simulink model "hostpc_can"  (Simulink 7.3)
settings: Solver=VariableStepDiscrete  StartTime=0.0  StopTime=inf  RelTol=1e-3
libraries: simulink x33, amg_usbconverter_n_connect_lib x3
settings Model: Creator=Nav  LastModifiedBy=Nav

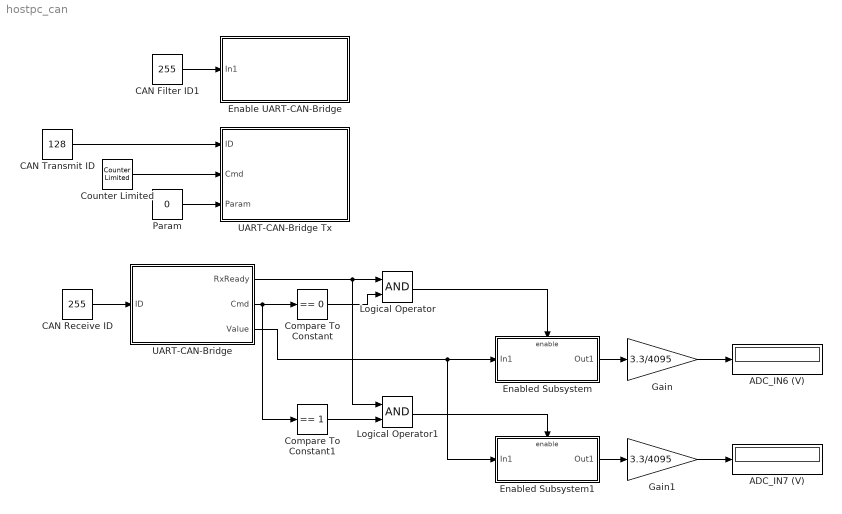
== system hostpc_can ==
  ADC_IN6 (V) : Display
  ADC_IN7 (V) : Display
  CAN Filter ID1 : Constant  Value=255  OutDataTypeMode=uint32  OutDataType=fixdt(1, 16)  OutScaling=2^0  OutDataTypeStr=uint32
  CAN Receive ID : Constant  Value=255  OutDataTypeMode=uint32  OutDataType=fixdt(1, 16)  OutScaling=2^0  OutDataTypeStr=uint32
  CAN Transmit ID : Constant  Value=128  OutDataTypeMode=uint32  OutDataType=fixdt(1, 16)  OutScaling=2^0  OutDataTypeStr=uint32
  Compare To Constant : simulink/Logic and Bit Operations/Compare To Constant  SystemSampleTime=-1  relop===  const=0  LogicOutDataTypeMode=boolean  ZeroCross=off
  Compare To Constant1 : simulink/Logic and Bit Operations/Compare To Constant  SystemSampleTime=-1  relop===  const=1  LogicOutDataTypeMode=boolean  ZeroCross=off
  Counter Limited : simulink/Sources/Counter Limited  SystemSampleTime=-1  uplimit=1  tsamp=-1
  Enable UART-CAN-Bridge : Subsystem  Priority=0
  Enabled Subsystem : Subsystem  TreatAsAtomicUnit=on
  Enabled Subsystem1 : Subsystem  TreatAsAtomicUnit=on
  Gain : Gain  Gain=3.3/4095  ParameterDataType=fixdt(1, 16)  ParameterScaling=2^0  OutDataType=fixdt(1, 16)  OutScaling=2^0
  Gain1 : Gain  Gain=3.3/4095  ParameterDataType=fixdt(1, 16)  ParameterScaling=2^0  OutDataType=fixdt(1, 16)  OutScaling=2^0
  Logical Operator : Logic  AllPortsSameDT=off  OutDataTypeMode=boolean  LogicDataType=fixdt(0, 8)  OutDataTypeStr=boolean
  Logical Operator1 : Logic  AllPortsSameDT=off  OutDataTypeMode=boolean  LogicDataType=fixdt(0, 8)  OutDataTypeStr=boolean
  Param : Constant  Value=0  OutDataTypeMode=uint32  OutDataType=fixdt(1, 16)  OutScaling=2^0  OutDataTypeStr=uint32
  UART-CAN-Bridge : Subsystem  Priority=2
  UART-CAN-Bridge Tx : Subsystem  Priority=1
  wires:
  CAN Receive ID/1 -> UART-CAN-Bridge/1(ID)
  CAN Transmit ID/1 -> UART-CAN-Bridge Tx/1(ID)
  Counter Limited/1 -> UART-CAN-Bridge Tx/2(Cmd)
  Param/1 -> UART-CAN-Bridge Tx/3(Param)
  UART-CAN-Bridge/2(Cmd) -> Compare To Constant/1, Compare To Constant1/1
  UART-CAN-Bridge/1(RxReady) -> Logical Operator/1, Logical Operator1/1
  Compare To Constant/1 -> Logical Operator/2
  Logical Operator/1 -> Enabled Subsystem/Enable
  UART-CAN-Bridge/3(Value) -> Enabled Subsystem/1(In1), Enabled Subsystem1/1(In1)
  Enabled Subsystem/1(Out1) -> Gain/1
  Logical Operator1/1 -> Enabled Subsystem1/Enable
  Compare To Constant1/1 -> Logical Operator1/2
  Enabled Subsystem1/1(Out1) -> Gain1/1
  CAN Filter ID1/1 -> Enable UART-CAN-Bridge/1(In1)
  Gain/1 -> ADC_IN6 (V)/1
  Gain1/1 -> ADC_IN7 (V)/1

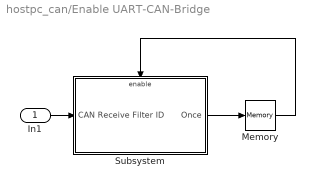
== system hostpc_can/Enable UART-CAN-Bridge ==
  In1 : Inport
  Memory : Memory  X0=1  InheritSampleTime=on  LinearizeMemory=on
  Subsystem : Subsystem
  wires:
  Subsystem/1(Once) -> Memory/1
  Memory/1 -> Subsystem/Enable
  In1/1 -> Subsystem/1(CAN Receive Filter ID)

== system hostpc_can/Enabled Subsystem ==
  In1 : Inport  OutDataType=fixdt(1, 16)  OutScaling=2^0
  Enable : EnablePort
  Out1 : Outport  OutDataType=fixdt(1, 16)  OutScaling=2^0
  wires:
  In1/1 -> Out1/1

== system hostpc_can/Enabled Subsystem1 ==
  In1 : Inport  OutDataType=fixdt(1, 16)  OutScaling=2^0
  Enable : EnablePort
  Out1 : Outport  OutDataType=fixdt(1, 16)  OutScaling=2^0
  wires:
  In1/1 -> Out1/1

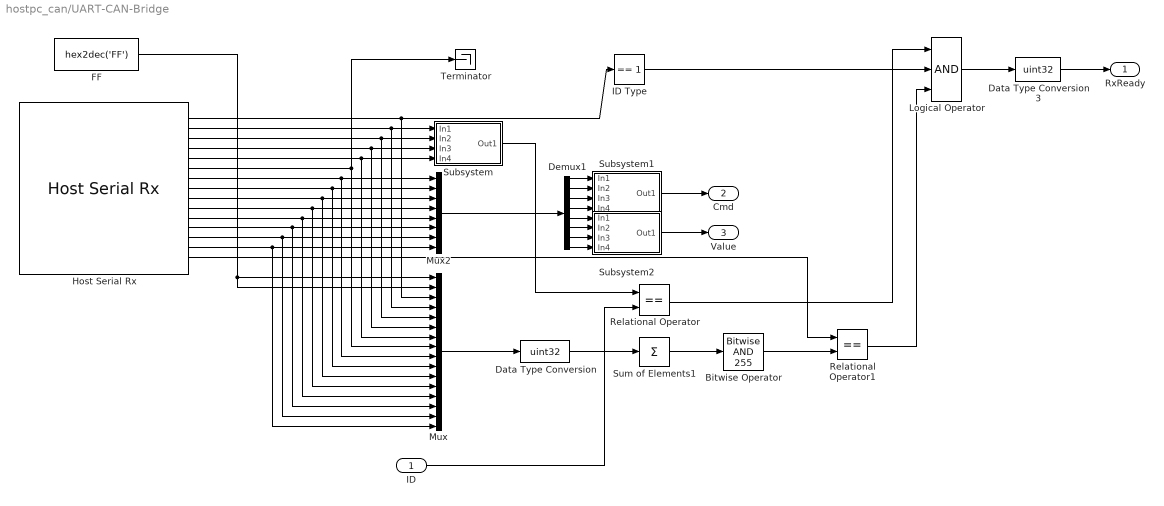
== system hostpc_can/UART-CAN-Bridge ==
  ID : Inport  OutDataType=fixdt(1, 16)  OutScaling=2^0
  Bitwise Operator : simulink/Logic and Bit Operations/Bitwise Operator  logicop=AND  UseBitMask=on  BitMask=255  BitMaskRealWorld=Stored Integer
  Data Type Conversion : DataTypeConversion  OutDataTypeMode=uint32  OutDataType=fixdt(1, 16)  OutScaling=2^0  OutDataTypeStr=uint32
  Data Type Conversion3 : DataTypeConversion  OutDataTypeMode=uint32  OutDataType=fixdt(1, 16)  OutScaling=2^0  OutDataTypeStr=uint32
  Demux1 : Demux  Outputs=8
  FF : Constant  Value=hex2dec('FF')  OutDataTypeMode=uint8  OutDataType=fixdt(1, 16)  OutScaling=2^0  OutDataTypeStr=uint8
  Host Serial Rx : amg_usbconverter_n_connect_lib/Host Serial Rx  conf=rx  port=<auto>  baudrate=115200  databits=8  parity=None  stopbit=1  flowcontrol=None  transfer=Blocking  timeout=2  packetmode=Binary  initialvalues=[0]  binheader='FF FF'  binterminator=''  porttype_double=0  porttype_single=0  porttype_int8=0  porttype_uint8=15  porttype_int16=0  porttype_uint16=0  porttype_int32=0  porttype_uint32=0  asciiformat='%d %u %x'  rx_asciiterminator="CRLF (0x0D 0x0A - \"\\r\\n\")"  tx_asciiterminator="CRLF (0x0D 0x0A - \"\\r\\n\")"  sampletime=inf  enablecustomportlabel=off  cinputportlabel=0  coutputportlabel=A  portpinstr=0  blockid=UARTCANBridgeHostSerialRx  inputporttype=[]  inputportwidth=[]  inputportlabel={}  outputporttype=[3 3 3 3 3 3 3 3 3 3 3 3 3 3 3]  outputportwidth=[1 1 1 1 1 1 1 1 1 1 1 1 1 1 1]  outputportlabel={'uint8','uint8','uint8','uint8','uint8','uint8','uint8','uint8','uint8','uint8','uint8','uint8','uint8','uint8','uint8'}  compat=0  optionstring="[\"Param1\",\"Param1\"]"  autoport='COM3'
  ID Type : simulink/Logic and Bit Operations/Compare To Constant  SystemSampleTime=-1  relop===  const=1  LogicOutDataTypeMode=uint8  ZeroCross=off
  Logical Operator : Logic  Inputs=3  AllPortsSameDT=off  OutDataTypeMode=boolean  LogicDataType=fixdt(0, 8)  OutDataTypeStr=boolean
  Mux : Mux  Inputs=16
  Mux2 : Mux  Inputs=8
  Relational Operator : RelationalOperator  Operator===  LogicOutDataTypeMode=boolean  LogicDataType=fixdt(0, 8)  OutDataTypeStr=boolean
  Relational Operator1 : RelationalOperator  Operator===  LogicOutDataTypeMode=boolean  LogicDataType=fixdt(0, 8)  OutDataTypeStr=boolean
  Subsystem : Subsystem
  Subsystem1 : Subsystem
  Subsystem2 : Subsystem
  Sum of Elements1 : Sum  Inputs=+  OutDataType=fixdt(1, 16)  OutScaling=2^-10
  Terminator : Terminator
  RxReady : Outport
  Cmd : Outport  Port=2
  Value : Outport  Port=3
  wires:
  Sum of Elements1/1 -> Bitwise Operator/1
  Host Serial Rx/15 -> Relational Operator1/1
  Mux/1 -> Data Type Conversion/1
  FF/1 -> Mux/2, Mux/1
  Subsystem/1(Out1) -> Relational Operator/1
  ID/1 -> Relational Operator/2
  Logical Operator/1 -> Data Type Conversion3/1
  Mux2/1 -> Demux1/1
  ID Type/1 -> Logical Operator/2
  Data Type Conversion/1 -> Sum of Elements1/1
  Bitwise Operator/1 -> Relational Operator1/2
  Host Serial Rx/1 -> ID Type/1, Mux/3
  Host Serial Rx/2 -> Subsystem/1(In1), Mux/4
  Host Serial Rx/3 -> Subsystem/2(In2), Mux/5
  Host Serial Rx/4 -> Subsystem/3(In3), Mux/6
  Host Serial Rx/5 -> Subsystem/4(In4), Mux/7
  Host Serial Rx/6 -> Terminator/1, Mux/8
  Host Serial Rx/7 -> Mux2/1, Mux/9
  Host Serial Rx/8 -> Mux2/2, Mux/10
  Host Serial Rx/9 -> Mux2/3, Mux/11
  Host Serial Rx/10 -> Mux2/4, Mux/12
  Host Serial Rx/11 -> Mux2/5, Mux/13
  Host Serial Rx/12 -> Mux2/6, Mux/14
  Host Serial Rx/13 -> Mux2/7, Mux/15
  Host Serial Rx/14 -> Mux2/8, Mux/16
  Relational Operator/1 -> Logical Operator/1
  Relational Operator1/1 -> Logical Operator/3
  Data Type Conversion3/1 -> RxReady/1
  Demux1/1 -> Subsystem1/1(In1)
  Demux1/2 -> Subsystem1/2(In2)
  Demux1/3 -> Subsystem1/3(In3)
  Demux1/4 -> Subsystem1/4(In4)
  Demux1/5 -> Subsystem2/1(In1)
  Demux1/6 -> Subsystem2/2(In2)
  Demux1/7 -> Subsystem2/3(In3)
  Demux1/8 -> Subsystem2/4(In4)
  Subsystem1/1(Out1) -> Cmd/1
  Subsystem2/1(Out1) -> Value/1

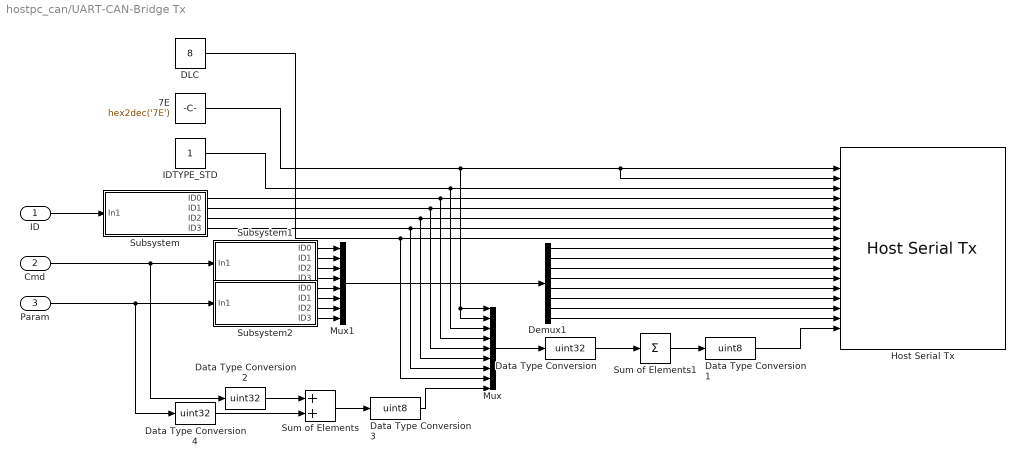
== system hostpc_can/UART-CAN-Bridge Tx ==
  ID : Inport
  Cmd : Inport  Port=2
  Param : Inport  Port=3
  7E : Constant  Value=hex2dec('7E')  OutDataTypeMode=uint8  OutDataType=fixdt(1, 16)  OutScaling=2^0  OutDataTypeStr=uint8
  DLC : Constant  Value=8  OutDataTypeMode=uint8  OutDataType=fixdt(1, 16)  OutScaling=2^0  OutDataTypeStr=uint8
  Data Type Conversion : DataTypeConversion  OutDataTypeMode=uint32  OutDataType=fixdt(1, 16)  OutScaling=2^0  OutDataTypeStr=uint32
  Data Type Conversion1 : DataTypeConversion  OutDataTypeMode=uint8  OutDataType=fixdt(1, 16)  OutScaling=2^0  OutDataTypeStr=uint8
  Data Type Conversion2 : DataTypeConversion  OutDataTypeMode=uint32  OutDataType=fixdt(1, 16)  OutScaling=2^0  OutDataTypeStr=uint32
  Data Type Conversion3 : DataTypeConversion  OutDataTypeMode=uint8  OutDataType=fixdt(1, 16)  OutScaling=2^0  OutDataTypeStr=uint8
  Data Type Conversion4 : DataTypeConversion  OutDataTypeMode=uint32  OutDataType=fixdt(1, 16)  OutScaling=2^0  OutDataTypeStr=uint32
  Demux1 : Demux  Outputs=8
  Host Serial Tx : amg_usbconverter_n_connect_lib/Host Serial Tx  conf=tx  port=<auto>  baudrate=115200  databits=8  parity=None  stopbit=1  flowcontrol=None  transfer=Blocking  timeout=2  packetmode=Binary  initialvalues=[]  binheader=''  binterminator=''  porttype_double=0  porttype_single=0  porttype_int8=0  porttype_uint8=17  porttype_int16=0  porttype_uint16=0  porttype_int32=0  porttype_uint32=0  asciiformat='%d %u %x'  rx_asciiterminator="CRLF (0x0D 0x0A - \"\\r\\n\")"  tx_asciiterminator="CRLF (0x0D 0x0A - \"\\r\\n\")"  sampletime=inf  enablecustomportlabel=off  cinputportlabel=0  coutputportlabel=A  portpinstr=0  blockid=UARTCANBridgeTxHostSerialTx  inputporttype=[3 3 3 3 3 3 3 3 3 3 3 3 3 3 3 3 3]  inputportwidth=[1 1 1 1 1 1 1 1 1 1 1 1 1 1 1 1 1]  inputportlabel={'uint8','uint8','uint8','uint8','uint8','uint8','uint8','uint8','uint8','uint8','uint8','uint8','uint8','uint8','uint8','uint8','uint8'}  outputporttype=[]  outputportwidth=[]  outputportlabel={}  compat=0  optionstring="[\"Param1\",\"Param1\"]"  autoport='COM3'
  IDTYPE_STD : Constant  OutDataTypeMode=uint8  OutDataType=fixdt(1, 16)  OutScaling=2^0  OutDataTypeStr=uint8
  Mux : Mux  Inputs=9
  Mux1 : Mux  Inputs=8
  Subsystem : Subsystem
  Subsystem1 : Subsystem
  Subsystem2 : Subsystem
  Sum of Elements : Sum  OutDataType=fixdt(1, 16)  OutScaling=2^-10
  Sum of Elements1 : Sum  Inputs=+  OutDataType=fixdt(1, 16)  OutScaling=2^-10
  wires:
  7E/1 -> Mux/1, Mux/2, Host Serial Tx/1, Host Serial Tx/2
  IDTYPE_STD/1 -> Host Serial Tx/3, Mux/3
  Subsystem/1(ID0) -> Host Serial Tx/4, Mux/4
  Subsystem/2(ID1) -> Host Serial Tx/5, Mux/5
  Subsystem/3(ID2) -> Host Serial Tx/6, Mux/6
  Subsystem/4(ID3) -> Host Serial Tx/7, Mux/7
  ID/1 -> Subsystem/1(In1)
  DLC/1 -> Host Serial Tx/8, Mux/8
  Demux1/1 -> Host Serial Tx/9
  Demux1/2 -> Host Serial Tx/10
  Demux1/3 -> Host Serial Tx/11
  Demux1/4 -> Host Serial Tx/12
  Demux1/5 -> Host Serial Tx/13
  Demux1/6 -> Host Serial Tx/14
  Demux1/7 -> Host Serial Tx/15
  Demux1/8 -> Host Serial Tx/16
  Sum of Elements/1 -> Data Type Conversion3/1
  Mux/1 -> Data Type Conversion/1
  Sum of Elements1/1 -> Data Type Conversion1/1
  Data Type Conversion/1 -> Sum of Elements1/1
  Data Type Conversion1/1 -> Host Serial Tx/17
  Data Type Conversion2/1 -> Sum of Elements/1
  Data Type Conversion3/1 -> Mux/9
  Mux1/1 -> Demux1/1
  Subsystem1/1(ID0) -> Mux1/1
  Subsystem1/2(ID1) -> Mux1/2
  Subsystem1/3(ID2) -> Mux1/3
  Subsystem1/4(ID3) -> Mux1/4
  Subsystem2/1(ID0) -> Mux1/5
  Subsystem2/2(ID1) -> Mux1/6
  Subsystem2/3(ID2) -> Mux1/7
  Subsystem2/4(ID3) -> Mux1/8
  Cmd/1 -> Subsystem1/1(In1), Data Type Conversion2/1
  Param/1 -> Subsystem2/1(In1), Data Type Conversion4/1
  Data Type Conversion4/1 -> Sum of Elements/2

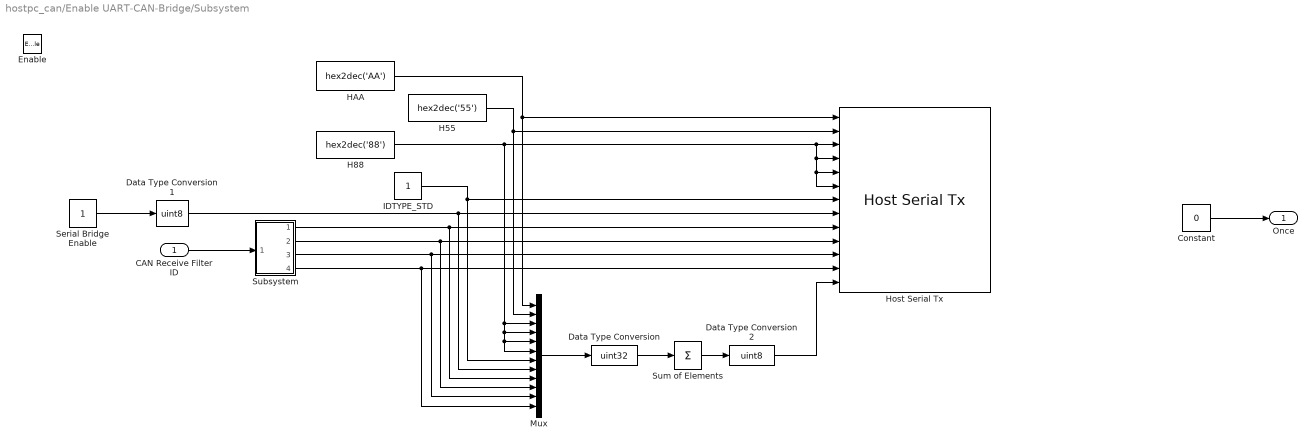
== system hostpc_can/Enable UART-CAN-Bridge/Subsystem ==
  CAN Receive Filter ID : Inport  OutDataType=fixdt(1, 16)  OutScaling=2^0
  Enable : EnablePort
  Constant : Constant  Value=0  OutDataType=fixdt(1, 16)  OutScaling=2^0
  Data Type Conversion : DataTypeConversion  OutDataTypeMode=uint32  OutDataType=fixdt(1, 16)  OutScaling=2^0  OutDataTypeStr=uint32
  Data Type Conversion1 : DataTypeConversion  OutDataTypeMode=uint8  OutDataType=fixdt(1, 16)  OutScaling=2^0  OutDataTypeStr=uint8
  Data Type Conversion2 : DataTypeConversion  OutDataTypeMode=uint8  OutDataType=fixdt(1, 16)  OutScaling=2^0  OutDataTypeStr=uint8
  H55 : Constant  Value=hex2dec('55')  OutDataTypeMode=uint8  OutDataType=fixdt(1, 16)  OutScaling=2^0  OutDataTypeStr=uint8
  H88 : Constant  Value=hex2dec('88')  OutDataTypeMode=uint8  OutDataType=fixdt(1, 16)  OutScaling=2^0  OutDataTypeStr=uint8
  HAA : Constant  Value=hex2dec('AA')  OutDataTypeMode=uint8  OutDataType=fixdt(1, 16)  OutScaling=2^0  OutDataTypeStr=uint8
  Host Serial Tx : amg_usbconverter_n_connect_lib/Host Serial Tx  conf=tx  port=<auto>  baudrate=115200  databits=8  parity=None  stopbit=1  flowcontrol=None  transfer=Blocking  timeout=2  packetmode=Binary  initialvalues=[]  binheader=''  binterminator=''  porttype_double=0  porttype_single=0  porttype_int8=0  porttype_uint8=13  porttype_int16=0  porttype_uint16=0  porttype_int32=0  porttype_uint32=0  asciiformat='%d %u %x'  rx_asciiterminator="CRLF (0x0D 0x0A - \"\\r\\n\")"  tx_asciiterminator="CRLF (0x0D 0x0A - \"\\r\\n\")"  sampletime=inf  enablecustomportlabel=off  cinputportlabel=0  coutputportlabel=A  portpinstr=0  blockid=EnableUARTCANBridgeSubsystemHostSerialTx  inputporttype=[3 3 3 3 3 3 3 3 3 3 3 3 3]  inputportwidth=[1 1 1 1 1 1 1 1 1 1 1 1 1]  inputportlabel={'uint8','uint8','uint8','uint8','uint8','uint8','uint8','uint8','uint8','uint8','uint8','uint8','uint8'}  outputporttype=[]  outputportwidth=[]  outputportlabel={}  compat=0  optionstring="[\"Param1\",\"Param1\"]"  autoport='COM3'
  IDTYPE_STD : Constant  OutDataTypeMode=uint8  OutDataType=fixdt(1, 16)  OutScaling=2^0  OutDataTypeStr=uint8
  Mux : Mux  Inputs=12
  Serial Bridge Enable : Constant  OutDataTypeMode=uint8  OutDataType=fixdt(1, 16)  OutScaling=2^0  OutDataTypeStr=uint8
  Subsystem : Subsystem
  Sum of Elements : Sum  Inputs=+  OutDataType=fixdt(1, 16)  OutScaling=2^-10
  Once : Outport  OutDataType=fixdt(1, 16)  OutScaling=2^0  InitialOutput=1
  wires:
  Serial Bridge Enable/1 -> Data Type Conversion1/1
  HAA/1 -> Host Serial Tx/1, Mux/1
  H55/1 -> Host Serial Tx/2, Mux/2
  IDTYPE_STD/1 -> Host Serial Tx/7, Mux/7
  Data Type Conversion1/1 -> Host Serial Tx/8, Mux/8
  Mux/1 -> Data Type Conversion/1
  Sum of Elements/1 -> Data Type Conversion2/1
  Data Type Conversion/1 -> Sum of Elements/1
  Data Type Conversion2/1 -> Host Serial Tx/13
  H88/1 -> Host Serial Tx/3, Host Serial Tx/4, Host Serial Tx/5, Host Serial Tx/6, Mux/3, Mux/4, Mux/5, Mux/6
  Subsystem/1(Out1) -> Host Serial Tx/9, Mux/9
  Subsystem/2(Out2) -> Host Serial Tx/10, Mux/10
  Subsystem/3(Out3) -> Host Serial Tx/11, Mux/11
  Subsystem/4(Out4) -> Host Serial Tx/12, Mux/12
  CAN Receive Filter ID/1 -> Subsystem/1(In1)
  Constant/1 -> Once/1

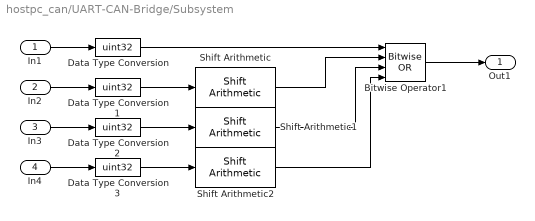
== system hostpc_can/UART-CAN-Bridge/Subsystem ==
  In1 : Inport  OutDataType=fixdt(1, 16)  OutScaling=2^0
  In2 : Inport  Port=2  OutDataType=fixdt(1, 16)  OutScaling=2^0
  In3 : Inport  Port=3  OutDataType=fixdt(1, 16)  OutScaling=2^0
  In4 : Inport  Port=4  OutDataType=fixdt(1, 16)  OutScaling=2^0
  Bitwise Operator1 : simulink/Logic and Bit Operations/Bitwise Operator  logicop=OR  UseBitMask=off  NumInputPorts=4  BitMask=bin2dec('11011001')  BitMaskRealWorld=Stored Integer
  Data Type Conversion{,1..3} (4 alike) : DataTypeConversion  OutDataTypeMode=uint32  OutDataType=fixdt(1, 16)  OutScaling=2^0  OutDataTypeStr=uint32
  Shift Arithmetic : simulink/Logic and Bit Operations/Shift Arithmetic  SystemSampleTime=-1  nBitShiftRight=-8  nBinPtShiftRight=0
  Shift Arithmetic1 : simulink/Logic and Bit Operations/Shift Arithmetic  SystemSampleTime=-1  nBitShiftRight=-16  nBinPtShiftRight=0
  Shift Arithmetic2 : simulink/Logic and Bit Operations/Shift Arithmetic  SystemSampleTime=-1  nBitShiftRight=-24  nBinPtShiftRight=0
  Out1 : Outport  OutDataType=fixdt(1, 16)  OutScaling=2^0
  wires:
  Bitwise Operator1/1 -> Out1/1
  Shift Arithmetic2/1 -> Bitwise Operator1/4
  Shift Arithmetic1/1 -> Bitwise Operator1/3
  Shift Arithmetic/1 -> Bitwise Operator1/2
  Data Type Conversion/1 -> Bitwise Operator1/1
  Data Type Conversion3/1 -> Shift Arithmetic2/1
  Data Type Conversion2/1 -> Shift Arithmetic1/1
  Data Type Conversion1/1 -> Shift Arithmetic/1
  In4/1 -> Data Type Conversion3/1
  In3/1 -> Data Type Conversion2/1
  In2/1 -> Data Type Conversion1/1
  In1/1 -> Data Type Conversion/1

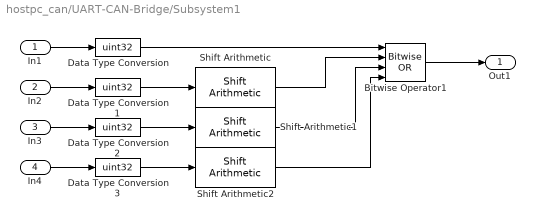
== system hostpc_can/UART-CAN-Bridge/Subsystem1 ==
  In1 : Inport  OutDataType=fixdt(1, 16)  OutScaling=2^0
  In2 : Inport  Port=2  OutDataType=fixdt(1, 16)  OutScaling=2^0
  In3 : Inport  Port=3  OutDataType=fixdt(1, 16)  OutScaling=2^0
  In4 : Inport  Port=4  OutDataType=fixdt(1, 16)  OutScaling=2^0
  Bitwise Operator1 : simulink/Logic and Bit Operations/Bitwise Operator  logicop=OR  UseBitMask=off  NumInputPorts=4  BitMask=bin2dec('11011001')  BitMaskRealWorld=Stored Integer
  Data Type Conversion{,1..3} (4 alike) : DataTypeConversion  OutDataTypeMode=uint32  OutDataType=fixdt(1, 16)  OutScaling=2^0  OutDataTypeStr=uint32
  Shift Arithmetic : simulink/Logic and Bit Operations/Shift Arithmetic  SystemSampleTime=-1  nBitShiftRight=-8  nBinPtShiftRight=0
  Shift Arithmetic1 : simulink/Logic and Bit Operations/Shift Arithmetic  SystemSampleTime=-1  nBitShiftRight=-16  nBinPtShiftRight=0
  Shift Arithmetic2 : simulink/Logic and Bit Operations/Shift Arithmetic  SystemSampleTime=-1  nBitShiftRight=-24  nBinPtShiftRight=0
  Out1 : Outport  OutDataType=fixdt(1, 16)  OutScaling=2^0
  wires:
  In1/1 -> Data Type Conversion/1
  In2/1 -> Data Type Conversion1/1
  In3/1 -> Data Type Conversion2/1
  In4/1 -> Data Type Conversion3/1
  Data Type Conversion1/1 -> Shift Arithmetic/1
  Data Type Conversion2/1 -> Shift Arithmetic1/1
  Data Type Conversion3/1 -> Shift Arithmetic2/1
  Data Type Conversion/1 -> Bitwise Operator1/1
  Shift Arithmetic/1 -> Bitwise Operator1/2
  Shift Arithmetic1/1 -> Bitwise Operator1/3
  Shift Arithmetic2/1 -> Bitwise Operator1/4
  Bitwise Operator1/1 -> Out1/1

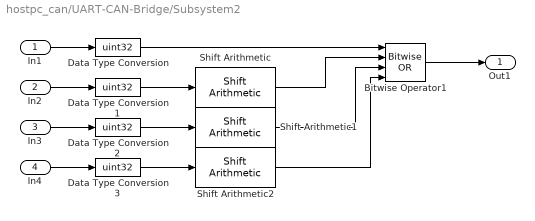
== system hostpc_can/UART-CAN-Bridge/Subsystem2 ==
  In1 : Inport  OutDataType=fixdt(1, 16)  OutScaling=2^0
  In2 : Inport  Port=2  OutDataType=fixdt(1, 16)  OutScaling=2^0
  In3 : Inport  Port=3  OutDataType=fixdt(1, 16)  OutScaling=2^0
  In4 : Inport  Port=4  OutDataType=fixdt(1, 16)  OutScaling=2^0
  Bitwise Operator1 : simulink/Logic and Bit Operations/Bitwise Operator  logicop=OR  UseBitMask=off  NumInputPorts=4  BitMask=bin2dec('11011001')  BitMaskRealWorld=Stored Integer
  Data Type Conversion{,1..3} (4 alike) : DataTypeConversion  OutDataTypeMode=uint32  OutDataType=fixdt(1, 16)  OutScaling=2^0  OutDataTypeStr=uint32
  Shift Arithmetic : simulink/Logic and Bit Operations/Shift Arithmetic  SystemSampleTime=-1  nBitShiftRight=-8  nBinPtShiftRight=0
  Shift Arithmetic1 : simulink/Logic and Bit Operations/Shift Arithmetic  SystemSampleTime=-1  nBitShiftRight=-16  nBinPtShiftRight=0
  Shift Arithmetic2 : simulink/Logic and Bit Operations/Shift Arithmetic  SystemSampleTime=-1  nBitShiftRight=-24  nBinPtShiftRight=0
  Out1 : Outport  OutDataType=fixdt(1, 16)  OutScaling=2^0
  wires:
  Bitwise Operator1/1 -> Out1/1
  Shift Arithmetic2/1 -> Bitwise Operator1/4
  Shift Arithmetic1/1 -> Bitwise Operator1/3
  Shift Arithmetic/1 -> Bitwise Operator1/2
  Data Type Conversion/1 -> Bitwise Operator1/1
  Data Type Conversion3/1 -> Shift Arithmetic2/1
  Data Type Conversion2/1 -> Shift Arithmetic1/1
  Data Type Conversion1/1 -> Shift Arithmetic/1
  In4/1 -> Data Type Conversion3/1
  In3/1 -> Data Type Conversion2/1
  In2/1 -> Data Type Conversion1/1
  In1/1 -> Data Type Conversion/1

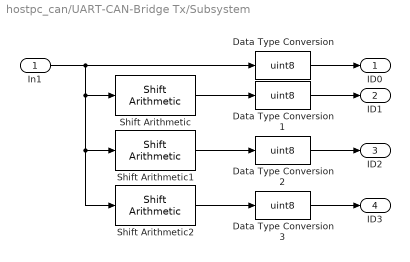
== system hostpc_can/UART-CAN-Bridge Tx/Subsystem ==
  In1 : Inport  OutDataType=fixdt(1, 16)  OutScaling=2^0
  Data Type Conversion{,1..3} (4 alike) : DataTypeConversion  OutDataTypeMode=uint8  OutDataType=fixdt(1, 16)  OutScaling=2^0  OutDataTypeStr=uint8
  Shift Arithmetic : simulink/Logic and Bit Operations/Shift Arithmetic  SystemSampleTime=-1  nBitShiftRight=8  nBinPtShiftRight=0
  Shift Arithmetic1 : simulink/Logic and Bit Operations/Shift Arithmetic  SystemSampleTime=-1  nBitShiftRight=16  nBinPtShiftRight=0
  Shift Arithmetic2 : simulink/Logic and Bit Operations/Shift Arithmetic  SystemSampleTime=-1  nBitShiftRight=24  nBinPtShiftRight=0
  ID0 : Outport  OutDataType=fixdt(1, 16)  OutScaling=2^0
  ID1 : Outport  Port=2  OutDataType=fixdt(1, 16)  OutScaling=2^0
  ID2 : Outport  Port=3  OutDataType=fixdt(1, 16)  OutScaling=2^0
  ID3 : Outport  Port=4  OutDataType=fixdt(1, 16)  OutScaling=2^0
  wires:
  In1/1 -> Data Type Conversion/1, Shift Arithmetic/1, Shift Arithmetic1/1, Shift Arithmetic2/1
  Data Type Conversion/1 -> ID0/1
  Shift Arithmetic/1 -> Data Type Conversion1/1
  Shift Arithmetic1/1 -> Data Type Conversion2/1
  Shift Arithmetic2/1 -> Data Type Conversion3/1
  Data Type Conversion1/1 -> ID1/1
  Data Type Conversion2/1 -> ID2/1
  Data Type Conversion3/1 -> ID3/1

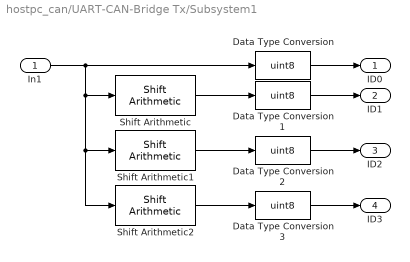
== system hostpc_can/UART-CAN-Bridge Tx/Subsystem1 ==
  In1 : Inport  OutDataType=fixdt(1, 16)  OutScaling=2^0
  Data Type Conversion{,1..3} (4 alike) : DataTypeConversion  OutDataTypeMode=uint8  OutDataType=fixdt(1, 16)  OutScaling=2^0  OutDataTypeStr=uint8
  Shift Arithmetic : simulink/Logic and Bit Operations/Shift Arithmetic  SystemSampleTime=-1  nBitShiftRight=8  nBinPtShiftRight=0
  Shift Arithmetic1 : simulink/Logic and Bit Operations/Shift Arithmetic  SystemSampleTime=-1  nBitShiftRight=16  nBinPtShiftRight=0
  Shift Arithmetic2 : simulink/Logic and Bit Operations/Shift Arithmetic  SystemSampleTime=-1  nBitShiftRight=24  nBinPtShiftRight=0
  ID0 : Outport  OutDataType=fixdt(1, 16)  OutScaling=2^0
  ID1 : Outport  Port=2  OutDataType=fixdt(1, 16)  OutScaling=2^0
  ID2 : Outport  Port=3  OutDataType=fixdt(1, 16)  OutScaling=2^0
  ID3 : Outport  Port=4  OutDataType=fixdt(1, 16)  OutScaling=2^0
  wires:
  Data Type Conversion3/1 -> ID3/1
  Data Type Conversion2/1 -> ID2/1
  Data Type Conversion1/1 -> ID1/1
  Shift Arithmetic2/1 -> Data Type Conversion3/1
  Shift Arithmetic1/1 -> Data Type Conversion2/1
  Shift Arithmetic/1 -> Data Type Conversion1/1
  Data Type Conversion/1 -> ID0/1
  In1/1 -> Shift Arithmetic2/1, Shift Arithmetic1/1, Shift Arithmetic/1, Data Type Conversion/1

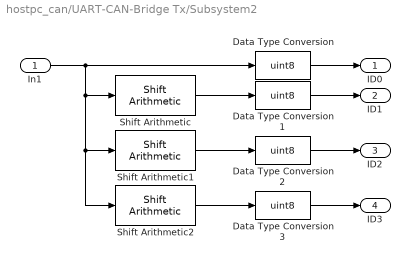
== system hostpc_can/UART-CAN-Bridge Tx/Subsystem2 ==
  In1 : Inport  OutDataType=fixdt(1, 16)  OutScaling=2^0
  Data Type Conversion{,1..3} (4 alike) : DataTypeConversion  OutDataTypeMode=uint8  OutDataType=fixdt(1, 16)  OutScaling=2^0  OutDataTypeStr=uint8
  Shift Arithmetic : simulink/Logic and Bit Operations/Shift Arithmetic  SystemSampleTime=-1  nBitShiftRight=8  nBinPtShiftRight=0
  Shift Arithmetic1 : simulink/Logic and Bit Operations/Shift Arithmetic  SystemSampleTime=-1  nBitShiftRight=16  nBinPtShiftRight=0
  Shift Arithmetic2 : simulink/Logic and Bit Operations/Shift Arithmetic  SystemSampleTime=-1  nBitShiftRight=24  nBinPtShiftRight=0
  ID0 : Outport  OutDataType=fixdt(1, 16)  OutScaling=2^0
  ID1 : Outport  Port=2  OutDataType=fixdt(1, 16)  OutScaling=2^0
  ID2 : Outport  Port=3  OutDataType=fixdt(1, 16)  OutScaling=2^0
  ID3 : Outport  Port=4  OutDataType=fixdt(1, 16)  OutScaling=2^0
  wires:
  In1/1 -> Data Type Conversion/1, Shift Arithmetic/1, Shift Arithmetic1/1, Shift Arithmetic2/1
  Data Type Conversion/1 -> ID0/1
  Shift Arithmetic/1 -> Data Type Conversion1/1
  Shift Arithmetic1/1 -> Data Type Conversion2/1
  Shift Arithmetic2/1 -> Data Type Conversion3/1
  Data Type Conversion1/1 -> ID1/1
  Data Type Conversion2/1 -> ID2/1
  Data Type Conversion3/1 -> ID3/1

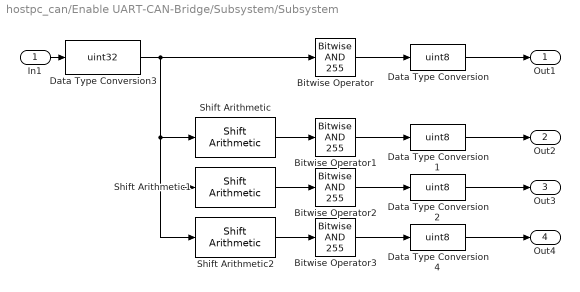
== system hostpc_can/Enable UART-CAN-Bridge/Subsystem/Subsystem ==
  In1 : Inport
  Bitwise Operator{,1..3} (4 alike) : simulink/Logic and Bit Operations/Bitwise Operator  logicop=AND  UseBitMask=on  BitMask=255  BitMaskRealWorld=Stored Integer
  Data Type Conversion{,1..2,4} (4 alike) : DataTypeConversion  OutDataTypeMode=uint8  OutDataType=fixdt(1, 16)  OutScaling=2^0  OutDataTypeStr=uint8
  Data Type Conversion3 : DataTypeConversion  OutDataTypeMode=uint32  OutDataType=fixdt(1, 16)  OutScaling=2^0  OutDataTypeStr=uint32
  Shift Arithmetic : simulink/Logic and Bit Operations/Shift Arithmetic  SystemSampleTime=-1  nBitShiftRight=8  nBinPtShiftRight=0
  Shift Arithmetic1 : simulink/Logic and Bit Operations/Shift Arithmetic  SystemSampleTime=-1  nBitShiftRight=16  nBinPtShiftRight=0
  Shift Arithmetic2 : simulink/Logic and Bit Operations/Shift Arithmetic  SystemSampleTime=-1  nBitShiftRight=24  nBinPtShiftRight=0
  Out1 : Outport
  Out2 : Outport  Port=2
  Out3 : Outport  Port=3
  Out4 : Outport  Port=4
  wires:
  Shift Arithmetic/1 -> Bitwise Operator1/1
  Shift Arithmetic1/1 -> Bitwise Operator2/1
  Shift Arithmetic2/1 -> Bitwise Operator3/1
  Data Type Conversion3/1 -> Bitwise Operator/1, Shift Arithmetic/1, Shift Arithmetic1/1, Shift Arithmetic2/1
  Bitwise Operator/1 -> Data Type Conversion/1
  In1/1 -> Data Type Conversion3/1
  Bitwise Operator1/1 -> Data Type Conversion1/1
  Bitwise Operator2/1 -> Data Type Conversion2/1
  Bitwise Operator3/1 -> Data Type Conversion4/1
  Data Type Conversion/1 -> Out1/1
  Data Type Conversion1/1 -> Out2/1
  Data Type Conversion2/1 -> Out3/1
  Data Type Conversion4/1 -> Out4/1
